simulink model "Example"  (R2022a)
settings: Solver=FixedStepDiscrete  StartTime=0.0  StopTime=60  RelTol=1e-3
values from neighbouring files (symbols this model uses):
  camMatrix = [1776.3684144  0  1044.42215992; 0  1886.39420352  628.091519225; 0  0  1]    [camMatrix.mat]
  distCoeff = [0.185126647266 -0.0224525942766 0.0197259842139 0.00469127635354]    [distCoeff.mat]
  markerSize = 0.105    [load_params.m]
undefined symbols (not defined in the file or in its folder): gray, Image, Mat, none, videoinput, x, y
libraries: opencvConverterBlockset x8, imaqlib x1, aruco_nano_detector_Lib x1
settings Model: Creator=Rafael  LastModifiedBy=Rafael
settings SFSimCC: SimTargetLang=C++

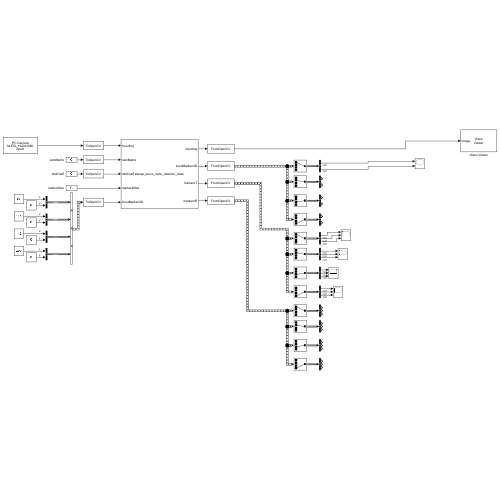
[thumbnail: Simulink's stored preview of the top-level diagram]
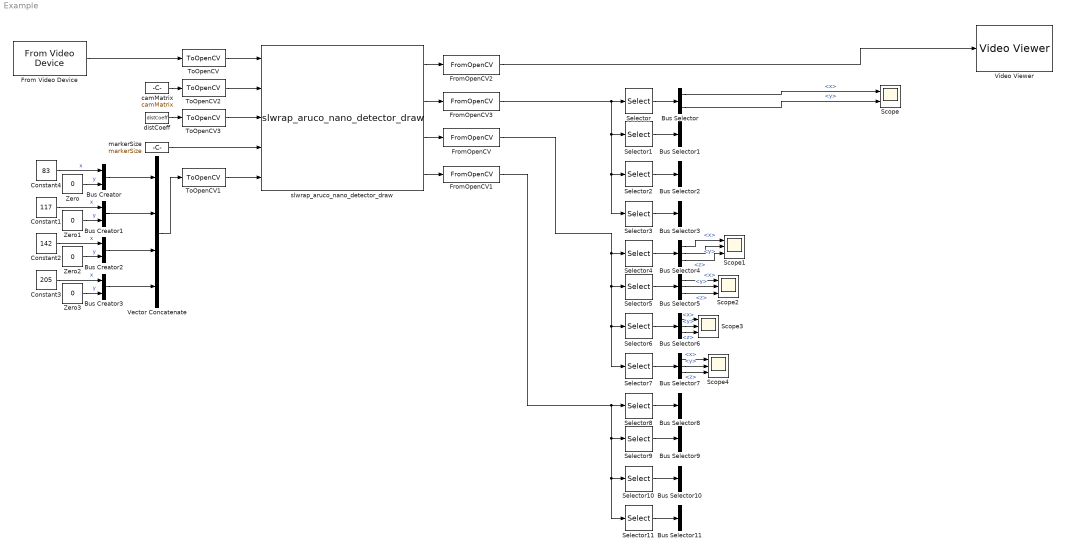
== system Example ==
  Bus Creator{,1..3} (4 alike) : BusCreator  Inputs=x,y  OutDataTypeStr=Bus: CV_POINT2I_BUS  NonVirtualBus=on
  Bus Selector{,1..3} (4 alike) : BusSelector  OutputSignals=x,y
  Bus Selector{4..11} (8 alike) : BusSelector  OutputSignals=x,y,z
  Constant1 : Constant  Value=117  OutDataTypeStr=int32
  Constant2 : Constant  Value=142  OutDataTypeStr=int32
  Constant3 : Constant  Value=205  OutDataTypeStr=int32
  Constant4 : Constant  Value=83  OutDataTypeStr=int32
  From Video Device : imaqlib/From Video Device  DeviceMenu=winvideo 1 (PC Camera)  Device=winvideo 1 (PC Camera)  ObjConstructor=videoinput('winvideo', 1)  VideoFormatMenu=MJPG_1920x1080  VideoFormat=MJPG_1920x1080  VideoSource=input1  ROIPosition=[0 0 1080 1920]  EnableHWTrigger=off  TriggerConfiguration=none/none  SampleTime=1/10  OutputPortsMode=One multidimensional signal  DataType=uint8  CanDoHWTrigger=no  ReturnedColorSpace=rgb  BlockHandle=4.0006  ROIWidth=1920  ROIHeight=1080  ROIColumn=0  ROIRow=0  EngXMLPath=C:\Program Files\MATLAB\R2022a\toolbox\imaq\imaq\private  DevXMLPath=C:\ProgramData\MATLAB\SupportPackages\R2022a\toolbox\imaq\supportpackages\genericvideo\adaptor\win64  EngLibPath=C:\Program Files\MATLAB\R2022a\toolbox\imaq\imaqblks\imaqmex\win64  ColorSpace=rgb  BayerSensorAlignment=grbg  ImaqMode=off
  FromOpenCV : opencvConverterBlockset/FromOpenCV  dataType=vector<Point3d>  rows=4  columns=1  channels=1  underlyingDataType=uint8  arrayLayout=Column-major  colorFormat=RGB
      settings: SourceProductBaseCode=SM_OPENCV
  FromOpenCV1 : opencvConverterBlockset/FromOpenCV  dataType=vector<Point3d>  rows=4  columns=1  channels=1  underlyingDataType=uint8  arrayLayout=Column-major  colorFormat=RGB
      settings: SourceProductBaseCode=SM_OPENCV
  FromOpenCV2 : opencvConverterBlockset/FromOpenCV  dataType=Mat-Image  rows=1080  columns=1920  channels=3  underlyingDataType=uint8  arrayLayout=Column-major  colorFormat=RGB
      settings: SourceProductBaseCode=SM_OPENCV
  FromOpenCV3 : opencvConverterBlockset/FromOpenCV  dataType=vector<Point2i>  rows=4  columns=1  channels=1  underlyingDataType=uint8  arrayLayout=Column-major  colorFormat=RGB
      settings: SourceProductBaseCode=SM_OPENCV
  Scope : Scope  NumInputPorts=2
  Scope{1..4} (4 alike) : Scope  NumInputPorts=3
  Selector : Selector  InputPortWidth=4  IndexOptions=Index vector (dialog)  Indices=[1]  OutputSizes=1
  Selector1 : Selector  InputPortWidth=4  IndexOptions=Index vector (dialog)  Indices=[2]  OutputSizes=1
  Selector10 : Selector  InputPortWidth=4  IndexOptions=Index vector (dialog)  Indices=[3]  OutputSizes=1
  Selector11 : Selector  InputPortWidth=4  IndexOptions=Index vector (dialog)  Indices=[4]  OutputSizes=1
  Selector2 : Selector  InputPortWidth=4  IndexOptions=Index vector (dialog)  Indices=[3]  OutputSizes=1
  Selector3 : Selector  InputPortWidth=4  IndexOptions=Index vector (dialog)  Indices=[4]  OutputSizes=1
  Selector4 : Selector  InputPortWidth=4  IndexOptions=Index vector (dialog)  Indices=[1]  OutputSizes=1
  Selector5 : Selector  InputPortWidth=4  IndexOptions=Index vector (dialog)  Indices=[2]  OutputSizes=1
  Selector6 : Selector  InputPortWidth=4  IndexOptions=Index vector (dialog)  Indices=[3]  OutputSizes=1
  Selector7 : Selector  InputPortWidth=4  IndexOptions=Index vector (dialog)  Indices=[4]  OutputSizes=1
  Selector8 : Selector  InputPortWidth=4  IndexOptions=Index vector (dialog)  Indices=[1]  OutputSizes=1
  Selector9 : Selector  InputPortWidth=4  IndexOptions=Index vector (dialog)  Indices=[2]  OutputSizes=1
  ToOpenCV : opencvConverterBlockset/ToOpenCV  dataType=Mat-Image
      settings: SourceProductBaseCode=SM_OPENCV
  ToOpenCV1 : opencvConverterBlockset/ToOpenCV  dataType=vector<Point2i>
      settings: SourceProductBaseCode=SM_OPENCV
  ToOpenCV2 : opencvConverterBlockset/ToOpenCV  dataType=Mat-Image
      settings: SourceProductBaseCode=SM_OPENCV
  ToOpenCV3 : opencvConverterBlockset/ToOpenCV  dataType=Mat
      settings: SourceProductBaseCode=SM_OPENCV
  Vector Concatenate : Concatenate  NumInputs=4
  Video Viewer : VideoViewer  colormapValue=gray(256)  FigPos=[1 814 1536 716]
  Zero{,1..3} (4 alike) : Constant  Value=0  OutDataTypeStr=int32
  camMatrix : Constant  Value=camMatrix
  distCoeff : Constant  Value=distCoeff  VectorParams1D=off
  markerSize : Constant  Value=markerSize
  slwrap_aruco_nano_detector_draw : aruco_nano_detector_Lib/slwrap_aruco_nano_detector_draw
  wires:
  FromOpenCV2/1 -> Video Viewer/1
  From Video Device/1 -> ToOpenCV/1
  Bus Creator/1 -> Vector Concatenate/1
  camMatrix/1 -> ToOpenCV2/1
  distCoeff/1 -> ToOpenCV3/1
  Constant4/1 -> Bus Creator/1  "x"
  Zero/1 -> Bus Creator/2  "y"
  slwrap_aruco_nano_detector_draw/3 -> FromOpenCV/1
  ToOpenCV/1 -> slwrap_aruco_nano_detector_draw/1
  slwrap_aruco_nano_detector_draw/1 -> FromOpenCV2/1
  slwrap_aruco_nano_detector_draw/4 -> FromOpenCV1/1
  ToOpenCV2/1 -> slwrap_aruco_nano_detector_draw/2
  slwrap_aruco_nano_detector_draw/2 -> FromOpenCV3/1
  ToOpenCV1/1 -> slwrap_aruco_nano_detector_draw/5
  markerSize/1 -> slwrap_aruco_nano_detector_draw/4
  ToOpenCV3/1 -> slwrap_aruco_nano_detector_draw/3
  Vector Concatenate/1 -> ToOpenCV1/1
  Constant1/1 -> Bus Creator1/1  "x"
  Zero1/1 -> Bus Creator1/2  "y"
  Bus Creator1/1 -> Vector Concatenate/2
  Constant2/1 -> Bus Creator2/1  "x"
  Zero2/1 -> Bus Creator2/2  "y"
  Bus Creator2/1 -> Vector Concatenate/3
  Constant3/1 -> Bus Creator3/1  "x"
  Zero3/1 -> Bus Creator3/2  "y"
  Bus Creator3/1 -> Vector Concatenate/4
  Selector/1 -> Bus Selector/1
  Selector1/1 -> Bus Selector1/1
  Selector2/1 -> Bus Selector2/1
  Selector3/1 -> Bus Selector3/1
  FromOpenCV3/1 -> Selector3/1, Selector2/1, Selector1/1, Selector/1
  FromOpenCV/1 -> Selector7/1, Selector6/1, Selector5/1, Selector4/1
  FromOpenCV1/1 -> Selector11/1, Selector10/1, Selector9/1, Selector8/1
  Selector4/1 -> Bus Selector4/1
  Selector5/1 -> Bus Selector5/1
  Selector6/1 -> Bus Selector6/1
  Selector7/1 -> Bus Selector7/1
  Selector8/1 -> Bus Selector8/1
  Selector9/1 -> Bus Selector9/1
  Selector10/1 -> Bus Selector10/1
  Selector11/1 -> Bus Selector11/1
  Bus Selector/2 -> Scope/2  "<y>"
  Bus Selector/1 -> Scope/1  "<x>"
  Bus Selector4/1 -> Scope1/1  "<x>"
  Bus Selector4/2 -> Scope1/2  "<y>"
  Bus Selector4/3 -> Scope1/3  "<z>"
  Bus Selector5/2 -> Scope2/2  "<y>"
  Bus Selector5/1 -> Scope2/1  "<x>"
  Bus Selector5/3 -> Scope2/3  "<z>"
  Bus Selector6/1 -> Scope3/1  "<x>"
  Bus Selector6/2 -> Scope3/2  "<y>"
  Bus Selector6/3 -> Scope3/3  "<z>"
  Bus Selector7/1 -> Scope4/1  "<x>"
  Bus Selector7/2 -> Scope4/2  "<y>"
  Bus Selector7/3 -> Scope4/3  "<z>"
